simulink model "PEM_Fuelcell_Working Model"  (R2025b)
settings: Solver=VariableStepAuto  StartTime=0.0  StopTime=10  RelTol=1e-3
libraries: simulink x1
settings Model: Creator=User  LastModifiedBy=User

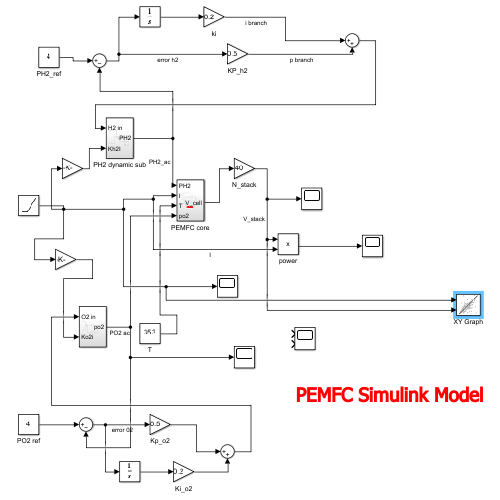
[thumbnail: Simulink's stored preview of the top-level diagram]
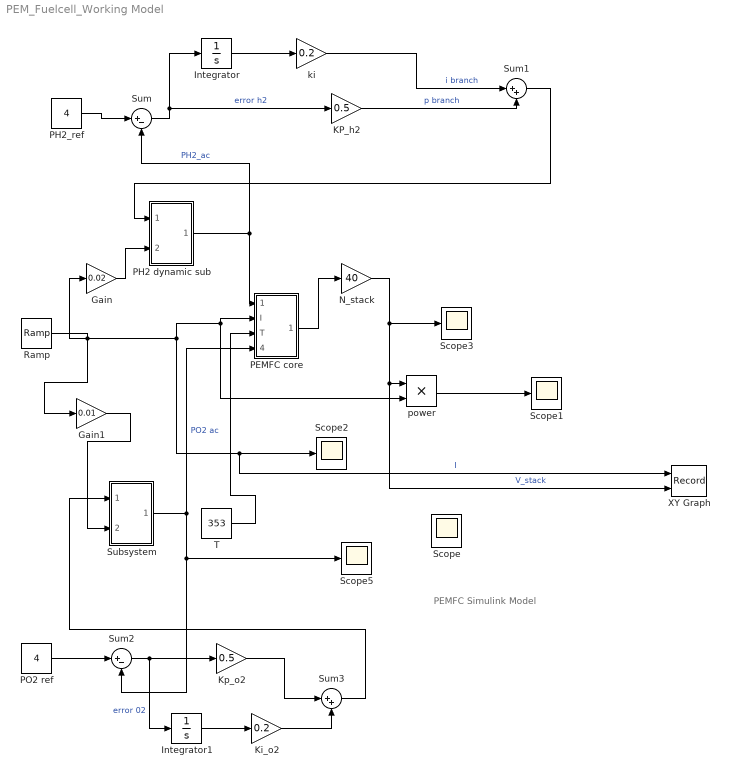
== system PEM_Fuelcell_Working Model ==
  note: PEMFC Simulink Model
  Gain : Gain  Gain=0.02
  Gain1 : Gain  Gain=0.01
  Integrator : Integrator
  Integrator1 : Integrator
  KP_h2 : Gain  Gain=0.5
  Ki_o2 : Gain  Gain=0.2
  Kp_o2 : Gain  Gain=0.5
  N_stack : Gain  Gain=40
  PEMFC core : Subsystem
  PH2 dynamic sub : Subsystem
  PH2_ref : Constant  Value=4
  PO2 ref : Constant  Value=4
  Ramp : simulink/Sources/Ramp  slope=1  start=0  InitialOutput=0
  Scope : Scope  NumInputPorts=2
      settings: ActiveDisplayYMinimum=-73.489535797221492  ActiveDisplayYMaximum=41.115939389988938
  Scope{1..3,5} (4 alike) : Scope
      Scope1 settings: ActiveDisplayYMinimum=20.53915211798838  ActiveDisplayYMaximum=234.76328482573271
      Scope2 settings: ActiveDisplayYMinimum=4.777201269955218  ActiveDisplayYMaximum=8.1785618141729053  DataLoggingVariableName=ScopeData2
      Scope3 settings: ActiveDisplayYMinimum=16.830410586307977  ActiveDisplayYMaximum=40.9758285682983  DataLoggingVariableName=ScopeData3
      Scope5 settings: ActiveDisplayYMinimum=2.5423384916992671  ActiveDisplayYMaximum=6.1528729641002364  DataLoggingVariableName=ScopeData5
  Subsystem : Subsystem
  Sum : Sum  Inputs=|+-
  Sum1 : Sum  Inputs=|++
  Sum2 : Sum  Inputs=|+-
  Sum3 : Sum  Inputs=|++
  T : Constant  Value=353
  XY Graph : Record  NumPorts=2.0  FileSettingsInternal="{\"entries\":[{\"content\":{\"excelSettings\":{\"content\":{},\"type\":\"Streamout.ExcelSettings\"},\"parquetSettings\":{\"content\":{},\"type\":\"Streamout.ParquetSettings\"}},\"type\":\"Streamout.FileSettingStorage\",\"uuid\":\"\"}],\"packageUris\":[\"http:\\/\\/schema.mathworks.com\\/mf0\\/streamout_blocks\\/R2020a\"],\"version\":\"1.0\"}"  FrameSettings=[0, 0]  Layout=[1 1]  SignalsInternal="{\"entries\":[{\"content\":{\"signals\":[{\"content\":{\"blockPath\":[],\"dimensions\":[1],\"domain\":\"\",\"lineColor\":\"#a2142f\",\"plots\":[ 1 ],\"port\":1,\"sid\":[\"\"],\"signalID\":1,\"signalName\":\"I\"},\"type\":\"RecordBlkView.Signal\",\"uuid\":\"\"},{\"content\":{\"blockPath\":[],\"dimensions\":[1],\"domain\":\"\",\"lineColor\":\"#139fff\",\"plots\":[ 1 ],\"port\":2,\"sid\":[\"\"],\"signalID\":2,\"signalName\":\"V_stack\"},\"type\":\"RecordBlkView.Signal\",\"uuid\":\"\"}]},\"type\":\"RecordBlkView.InputSignals\",\"uuid\":\"\"}],\"packageUris\":[\"http:\\/\\/schema.mathworks.com\\/mf0\\/streamout_blocks\\/R2020a\"],\"version\":\"1.0\"}"  VisualizationBindings="{\"xyplotplugin\":{\"info\":[{\"series\":[{\"bindingParametersList\":[{\"parameter\":\"X-Axis\",\"signalID\":1,\"signalName\":\"I\"},{\"parameter\":\"Y-Axis\",\"signalID\":2,\"signalName\":\"V_stack\"}],\"seriesID\":0}],\"subplotID\":1}]}}"  CompatibilityTag=XY
  ki : Gain  Gain=0.2
  power : Product
  wires:
  Ramp/1 -> power/2, PEMFC core/2(I), XY Graph/1, Scope2/1, Gain/1, Gain1/1  "I"
  T/1 -> PEMFC core/3(T)
  PEMFC core/1(V_cell) -> N_stack/1
  N_stack/1 -> Scope3/1, XY Graph/2, power/1  "V_stack"
  power/1 -> Scope1/1
  PH2 dynamic sub/1(PH2) -> PEMFC core/1(PH2), Sum/2  "PH2_ac"
  Gain1/1 -> Subsystem/2(Ko2i)
  Subsystem/1(po2) -> PEMFC core/4(po2), Scope5/1, Sum2/2  "PO2 ac"
  Gain/1 -> PH2 dynamic sub/2(Kh2I)
  PH2_ref/1 -> Sum/1
  Sum/1 -> Integrator/1, KP_h2/1  "error h2"
  Integrator/1 -> ki/1
  KP_h2/1 -> Sum1/2  "p branch"
  ki/1 -> Sum1/1  "i branch"
  Sum1/1 -> PH2 dynamic sub/1(H2 in)
  PO2 ref/1 -> Sum2/1
  Sum2/1 -> Integrator1/1, Kp_o2/1  "error 02"
  Integrator1/1 -> Ki_o2/1
  Ki_o2/1 -> Sum3/2
  Kp_o2/1 -> Sum3/1
  Sum3/1 -> Subsystem/1(O2 in)

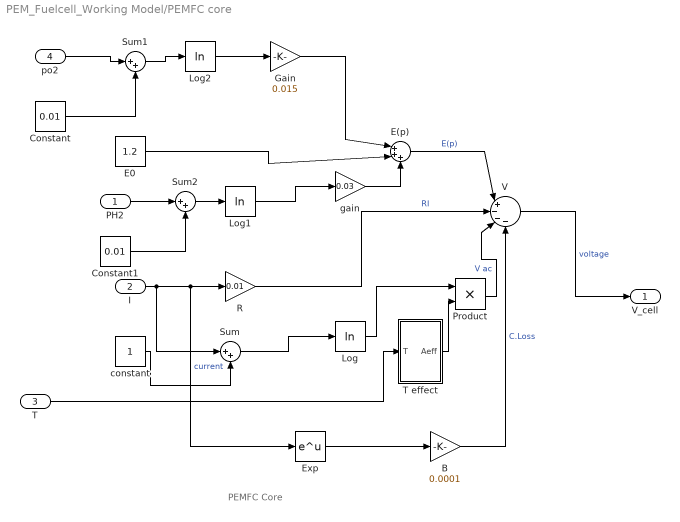
== system PEM_Fuelcell_Working Model/PEMFC core ==
  note: PEMFC Core
  PH2 : Inport
  I : Inport  Port=2
  T : Inport  Port=3
  po2 : Inport  Port=4
  B : Gain  Gain=0.0001
  Constant : Constant  Value=0.01
  Constant1 : Constant  Value=0.01
  E(p) : Sum  Inputs=|+++
  E0 : Constant  Value=1.2
  Exp : Math
  Gain : Gain  Gain=0.015
  Log : Math  Operator=log
  Log1 : Math  Operator=log
  Log2 : Math  Operator=log
  Product : Product
  R : Gain  Gain=0.01
  Sum : Sum  Inputs=|++
  Sum1 : Sum  Inputs=|++
  Sum2 : Sum  Inputs=|++
  T effect : Subsystem
  V : Sum  Inputs=|+---
  constant : Constant
  gain : Gain  Gain=0.03
  V_cell : Outport
  wires:
  V/1 -> V_cell/1  "voltage"
  I/1 -> Sum/1, Exp/1, R/1  "current"
  Sum/1 -> Log/1
  constant/1 -> Sum/2
  R/1 -> V/2  "RI"
  Log1/1 -> gain/1
  Exp/1 -> B/1
  E(p)/1 -> V/1  "E(p)"
  B/1 -> V/4  "C.Loss"
  T/1 -> T effect/1(T)
  Log/1 -> Product/1
  T effect/1(Aeff) -> Product/2
  Product/1 -> V/3  "V ac"
  po2/1 -> Sum1/1
  Log2/1 -> Gain/1
  gain/1 -> E(p)/3
  E0/1 -> E(p)/2
  Gain/1 -> E(p)/1
  Constant/1 -> Sum1/2
  Sum1/1 -> Log2/1
  PH2/1 -> Sum2/1
  Constant1/1 -> Sum2/2
  Sum2/1 -> Log1/1

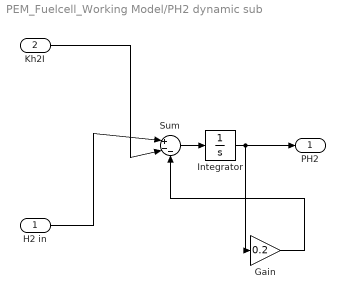
== system PEM_Fuelcell_Working Model/PH2 dynamic sub ==
  H2 in : Inport
  Kh2I : Inport  Port=2
  Gain : Gain  Gain=0.2
  Integrator : Integrator  InitialCondition=4
  Sum : Sum  Inputs=|+--
  PH2 : Outport
  wires:
  Sum/1 -> Integrator/1
  Integrator/1 -> Gain/1, PH2/1
  H2 in/1 -> Sum/1
  Kh2I/1 -> Sum/2
  Gain/1 -> Sum/3

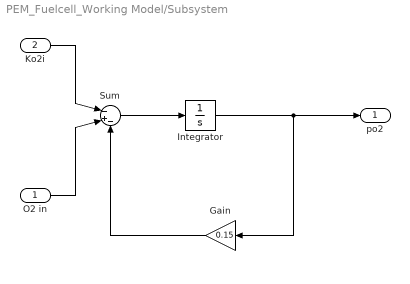
== system PEM_Fuelcell_Working Model/Subsystem ==
  O2 in : Inport
  Ko2i : Inport  Port=2
  Gain : Gain  Gain=0.15
  Integrator : Integrator  InitialCondition=4
  Sum : Sum  Inputs=|-+-
  po2 : Outport
  wires:
  O2 in/1 -> Sum/2
  Ko2i/1 -> Sum/1
  Sum/1 -> Integrator/1
  Integrator/1 -> Gain/1, po2/1
  Gain/1 -> Sum/3

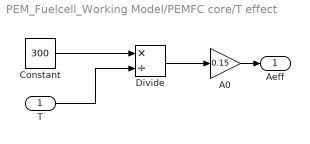
== system PEM_Fuelcell_Working Model/PEMFC core/T effect ==
  T : Inport
  A0 : Gain  Gain=0.15
  Constant : Constant  Value=300
  Divide : Product  Inputs=*/
  Aeff : Outport
  wires:
  Constant/1 -> Divide/1
  T/1 -> Divide/2
  Divide/1 -> A0/1
  A0/1 -> Aeff/1
